simulink library "myLibrary"  (R2023a)
settings: Solver=VariableStepAuto  StartTime=0.0  StopTime=10.0  RelTol=1e-3
undefined symbols (not defined in the file): Cac_n1, ctrl1, Da, Discrete, dtha, ee_sli_rtmsupport, FA, gcbh, Ha, Ini, init_line, init_load, init_SG, init_TH, init_trafo, init_VSC, initMachineBlocks, Ka, Lf, Llkd_pu, Llkq1_pu, NET, P, plots_step, q0, Rac_n1, Radd, Rkd_pu, Rkq1_pu, Rload_add, sim_config, spsSteamTurbineModel, T_global, T_load, T_NET, T_SG, T_TH, T_trafo, T_VSC, Ts, tstep, V1
libraries: spsSeriesRLCBranchLib x57, spsParallelRLCBranchLib x39, eeGeneralControl x38, spsCurrentMeasurementLib x20, spsFirstOrderFilterLib x16, spsVoltageMeasurementLib x14, spsControlledVoltageSourceLib x12, $bdroot x9, dspsigops x6, spsThreePhaseVIMeasurementLib x5, spsPLL3phLib x4, spsThreePhaseBreakerLib x3
(part 6 of 7)

== system myLibrary/SG_step/Governor-Turbine/Steam Turbine and Governor/Model/4 mass shaft/2 masses ==
  note: Eeach block Mass implements discretized state-space equations
      | of the shaft mass dynamics using trapezoidal method.
      |
      | x(k)= Ad*x(k-1) + Bd*(u(k)+u(k-1))
      |
      | where:
      | x(k) =  State vector = [dw_n             deltat_n   ]'
      | u(k) =  Input vector = [(Ts_n+1 + Tt_n)  deltat_n-1 ]'
      | n    =  Mass number
      |
      | % Discrete state-space matrices
      | Ad = inv(In - Ts/2*A)*(In + Ts/2*A)
      | Bd = inv(In - Ts/2*A)*B*Ts/2
      |
      | where:
      | Continuous state-space matrices:
      | A=[ -K1*D  -K1*K
      |      K2     0   ];
      |
      | B=[ K1  K1*K
      |      0     0];
      |
      | In = eye(2,2)
      | K  = Rigidity (pu)
      | K1 =1/(2*H);  H= inertia  (pu)
      | K2 =N*pi/30;  N=nominal speed of sync. machine (rpm)
  note: Mass1 = generator rotor simulated in synchronous machine model
  Tt_5-2 : Inport
  dth_gen : Inport  Port=2
  Enable : EnablePort  PropagateVarSize=During execution
  Demux : Demux  Outputs=2
      settings: DisplayOption=none
  Ground : Ground
  Ground1 : Ground
  Mass2 : Subsystem  mask(Generic rotating mass){H=Ha(1), K=Ka(1), D=Da(1), dth0=dtha(1), N=N, Ts=Ts}
      mask prompts: H "Inertia H (pu)"; K "Rigidity K (pu):"; D "Damping D (pu):"; dth0 "Initial angle deviation delta_theta (rad):"; N "Nominal speed of synchronous machine (rpm):"; Ts "Sample time (s):"
      mask init: same as myLibrary/SG/Governor-Turbine/Steam Turbine and Governor/Model/4 mass shaft/1 mass/Mass2
  Mass3 : Subsystem  mask(Generic rotating mass){H=Ha(2), K=Ka(2), D=Da(2), dth0=dtha(2), N=N, Ts=Ts}
      mask prompts: H "Inertia H (pu)"; K "Rigidity K (pu):"; D "Damping D (pu):"; dth0 "Initial angle deviation delta_theta (rad):"; N "Nominal speed of synchronous machine (rpm):"; Ts "Sample time (s):"
      mask init: same as myLibrary/SG/Governor-Turbine/Steam Turbine and Governor/Model/4 mass shaft/1 mass/Mass2
  Mux : Mux  Inputs=[ 2 1 1 ]
  Mux1 : Mux  Inputs=[ 2 1 1 ]
  Selector : Selector  InputPortWidth=4  IndexOptions=Index vector (dialog)  Indices=[3 4]  OutputSizes=1
  Terminator : Terminator
  Ts_5-2 : Outport  InitialOutput=[0,0,0,0]
  dw_5-2 : Outport  Port=2  InitialOutput=[0,0,0,0]
  Tm_gen : Outport  Port=3
  wires:
  Mass2/3(dw) -> Mux1/3
  Mass3/3(dw) -> Mux1/2
  Mux1/1 -> dw_5-2/1
  Ground1/1 -> Mux1/1, Mux/1
  Demux/1 -> Mass3/2(Tt_n)
  Tt_5-2/1 -> Selector/1
  Selector/1 -> Demux/1
  Mux/1 -> Ts_5-2/1
  Mass3/2("Ts_n ") -> Mux/2, Mass2/1(Ts_n+1)
  Mass3/1(deltat_n) -> Terminator/1
  Ground/1 -> Mass3/1(Ts_n+1)
  Demux/2 -> Mass2/2(Tt_n)
  Mass2/1(deltat_n) -> Mass3/3(deltat_n-1)
  dth_gen/1 -> Mass2/3(deltat_n-1)
  Mass2/2("Ts_n ") -> Mux/3, Tm_gen/1

== system myLibrary/SG_step/Governor-Turbine/Steam Turbine and Governor/Model/4 mass shaft/3 masses ==
  note: Eeach block Mass implements discretized state-space equations
      | of the shaft mass dynamics using trapezoidal method.
      |
      | x(k)= Ad*x(k-1) + Bd*(u(k)+u(k-1))
      |
      | where:
      | x(k) =  State vector = [dw_n             deltat_n   ]'
      | u(k) =  Input vector = [(Ts_n+1 + Tt_n)  deltat_n-1 ]'
      | n    =  Mass number
      |
      | % Discrete state-space matrices
      | Ad = inv(In - Ts/2*A)*(In + Ts/2*A)
      | Bd = inv(In - Ts/2*A)*B*Ts/2
      |
      | where:
      | Continuous state-space matrices:
      | A=[ -K1*D  -K1*K
      |      K2     0   ];
      |
      | B=[ K1  K1*K
      |      0     0];
      |
      | In = eye(2,2)
      | K  = Rigidity (pu)
      | K1 =1/(2*H);  H= inertia  (pu)
      | K2 =N*pi/30;  N=nominal speed of sync. machine (rpm)
  note: Mass1 = generator rotor simulated in synchronous machine model
  Tt_5-2 : Inport
  dth_gen : Inport  Port=2
  Enable : EnablePort  PropagateVarSize=During execution
  Demux : Demux  Outputs=3
      settings: DisplayOption=none
  Ground : Ground
  Ground1 : Ground
  Mass2 : Subsystem  mask(Generic rotating mass){H=Ha(1), K=Ka(1), D=Da(1), dth0=dtha(1), N=N, Ts=Ts}
      mask prompts: H "Inertia H (pu)"; K "Rigidity K (pu):"; D "Damping D (pu):"; dth0 "Initial angle deviation delta_theta (rad):"; N "Nominal speed of synchronous machine (rpm):"; Ts "Sample time (s):"
      mask init: same as myLibrary/SG/Governor-Turbine/Steam Turbine and Governor/Model/4 mass shaft/1 mass/Mass2
  Mass3 : Subsystem  mask(Generic rotating mass){H=Ha(2), K=Ka(2), D=Da(2), dth0=dtha(2), N=N, Ts=Ts}
      mask prompts: H "Inertia H (pu)"; K "Rigidity K (pu):"; D "Damping D (pu):"; dth0 "Initial angle deviation delta_theta (rad):"; N "Nominal speed of synchronous machine (rpm):"; Ts "Sample time (s):"
      mask init: same as myLibrary/SG/Governor-Turbine/Steam Turbine and Governor/Model/4 mass shaft/1 mass/Mass2
  Mass4 : Subsystem  mask(Generic rotating mass){H=Ha(3), K=Ka(3), D=Da(3), dth0=dtha(3), N=N, Ts=Ts}
      mask prompts: H "Inertia H (pu)"; K "Rigidity K (pu):"; D "Damping D (pu):"; dth0 "Initial angle deviation delta_theta (rad):"; N "Nominal speed of synchronous machine (rpm):"; Ts "Sample time (s):"
      mask init: same as myLibrary/SG/Governor-Turbine/Steam Turbine and Governor/Model/4 mass shaft/1 mass/Mass2
  Mux : Mux
  Mux1 : Mux
  Selector : Selector  InputPortWidth=4  IndexOptions=Index vector (dialog)  Indices=[2 3 4]  OutputSizes=1
  Terminator : Terminator
  Ts_5-2 : Outport  InitialOutput=[0,0,0,0]
  dw_5-2 : Outport  Port=2  InitialOutput=[0,0,0,0]
  Tm_gen : Outport  Port=3
  wires:
  Mass2/3(dw) -> Mux1/4
  Mux1/1 -> dw_5-2/1
  Ground1/1 -> Mux1/1, Mux/1
  Mux/1 -> Ts_5-2/1
  Mass3/3(dw) -> Mux1/3
  Mass4/3(dw) -> Mux1/2
  Mass4/2("Ts_n ") -> Mux/2, Mass3/1(Ts_n+1)
  Mass3/1(deltat_n) -> Mass4/3(deltat_n-1)
  Mass2/1(deltat_n) -> Mass3/3(deltat_n-1)
  Demux/3 -> Mass2/2(Tt_n)
  Demux/2 -> Mass3/2(Tt_n)
  Demux/1 -> Mass4/2(Tt_n)
  Ground/1 -> Mass4/1(Ts_n+1)
  Mass4/1(deltat_n) -> Terminator/1
  dth_gen/1 -> Mass2/3(deltat_n-1)
  Mass2/2("Ts_n ") -> Tm_gen/1, Mux/4
  Selector/1 -> Demux/1
  Tt_5-2/1 -> Selector/1
  Mass3/2("Ts_n ") -> Mux/3, Mass2/1(Ts_n+1)

== system myLibrary/SG_step/Governor-Turbine/Steam Turbine and Governor/Model/4 mass shaft/4 masses ==
  note: Eeach block Mass implements discretized state-space equations
      | of the shaft mass dynamics using trapezoidal method.
      |
      | x(k)= Ad*x(k-1) + Bd*(u(k)+u(k-1))
      |
      | where:
      | x(k) =  State vector = [dw_n             deltat_n   ]'
      | u(k) =  Input vector = [(Ts_n+1 + Tt_n)  deltat_n-1 ]'
      | n    =  Mass number
      |
      | % Discrete state-space matrices
      | Ad = inv(In - Ts/2*A)*(In + Ts/2*A)
      | Bd = inv(In - Ts/2*A)*B*Ts/2
      |
      | where:
      | Continuous state-space matrices:
      | A=[ -K1*D  -K1*K
      |      K2     0   ];
      |
      | B=[ K1  K1*K
      |      0     0];
      |
      | In = eye(2,2)
      | K  = Rigidity (pu)
      | K1 =1/(2*H);  H= inertia  (pu)
      | K2 =N*pi/30;  N=nominal speed of sync. machine (rpm)
  note: Mass1 = generator rotor simulated in synchronous machine model
  Tt_5-2 : Inport
  dth_gen : Inport  Port=2
  Enable : EnablePort  PropagateVarSize=During execution
  Demux : Demux
      settings: DisplayOption=none
  Ground : Ground
  Mass2 : Subsystem  mask(Generic rotating mass){H=Ha(1), K=Ka(1), D=Da(1), dth0=initSG.delta2, N=N, Ts=Ts}
      mask prompts: H "Inertia H (pu)"; K "Rigidity K (pu):"; D "Damping D (pu):"; dth0 "Initial angle deviation delta_theta (rad):"; N "Nominal speed of synchronous machine (rpm):"; Ts "Sample time (s):"
      mask init: same as myLibrary/SG/Governor-Turbine/Steam Turbine and Governor/Model/4 mass shaft/1 mass/Mass2
  Mass3 : Subsystem  mask(Generic rotating mass){H=Ha(2), K=Ka(2), D=Da(2), dth0=initSG.delta3, N=N, Ts=Ts}
      mask prompts: H "Inertia H (pu)"; K "Rigidity K (pu):"; D "Damping D (pu):"; dth0 "Initial angle deviation delta_theta (rad):"; N "Nominal speed of synchronous machine (rpm):"; Ts "Sample time (s):"
      mask init: same as myLibrary/SG/Governor-Turbine/Steam Turbine and Governor/Model/4 mass shaft/1 mass/Mass2
  Mass4 : Subsystem  mask(Generic rotating mass){H=Ha(3), K=Ka(3), D=Da(3), dth0=initSG.delta4, N=N, Ts=Ts}
      mask prompts: H "Inertia H (pu)"; K "Rigidity K (pu):"; D "Damping D (pu):"; dth0 "Initial angle deviation delta_theta (rad):"; N "Nominal speed of synchronous machine (rpm):"; Ts "Sample time (s):"
      mask init: same as myLibrary/SG/Governor-Turbine/Steam Turbine and Governor/Model/4 mass shaft/1 mass/Mass2
  Mass5 : Subsystem  mask(Generic rotating mass){H=Ha(4), K=Ka(4), D=Da(4), dth0=initSG.delta5, N=N, Ts=Ts}
      mask prompts: H "Inertia H (pu)"; K "Rigidity K (pu):"; D "Damping D (pu):"; dth0 "Initial angle deviation delta_theta (rad):"; N "Nominal speed of synchronous machine (rpm):"; Ts "Sample time (s):"
      mask init: same as myLibrary/SG/Governor-Turbine/Steam Turbine and Governor/Model/4 mass shaft/1 mass/Mass2
  Mux : Mux
  Mux1 : Mux
  Terminator : Terminator
  Ts_5-2 : Outport  InitialOutput=[0,0,0,0]
  dw_5-2 : Outport  Port=2  InitialOutput=[0,0,0,0]
  Tm_gen : Outport  Port=3
  wires:
  Mass2/3(dw) -> Mux1/4
  Mass3/3(dw) -> Mux1/3
  Mux1/1 -> dw_5-2/1
  Mass4/3(dw) -> Mux1/2
  Mass5/3(dw) -> Mux1/1
  Mux/1 -> Ts_5-2/1
  Mass5/1(deltat_n) -> Terminator/1
  Ground/1 -> Mass5/1(Ts_n+1)
  Demux/1 -> Mass5/2(Tt_n)
  Demux/2 -> Mass4/2(Tt_n)
  Demux/3 -> Mass3/2(Tt_n)
  Demux/4 -> Mass2/2(Tt_n)
  Mass2/1(deltat_n) -> Mass3/3(deltat_n-1)
  Mass3/1(deltat_n) -> Mass4/3(deltat_n-1)
  Mass4/1(deltat_n) -> Mass5/3(deltat_n-1)
  Mass5/2("Ts_n ") -> Mux/1, Mass4/1(Ts_n+1)
  Mass4/2("Ts_n ") -> Mux/2, Mass3/1(Ts_n+1)
  Mass3/2("Ts_n ") -> Mux/3, Mass2/1(Ts_n+1)
  Tt_5-2/1 -> Demux/1
  dth_gen/1 -> Mass2/3(deltat_n-1)
  Mass2/2("Ts_n ") -> Mux/4, Tm_gen/1

== system myLibrary/SG_step/Governor-Turbine/Steam Turbine and Governor/Model/steam turbine MM/Stage 1 ==
  In1 : Inport
  Constant4 : Constant  Value=Ta(1)~=0  SampleTime=Ts
  Stage1 : Subsystem  TreatAsAtomicUnit=on
  Switch : Switch  Threshold=0.5  SaturateOnIntegerOverflow=off
  Out1 : Outport
  wires:
  Constant4/1 -> Stage1/Enable, Switch/2
  In1/1 -> Stage1/1(In1), Switch/3
  Stage1/1(Out1) -> Switch/1
  Switch/1 -> Out1/1

== system myLibrary/SG_step/Governor-Turbine/Steam Turbine and Governor/Model/steam turbine MM/Stage 2  ==
  In1 : Inport
  Constant3 : Constant  Value=Ta(2)~=0  SampleTime=Ts
  Stage2 : Subsystem  TreatAsAtomicUnit=on
  Switch1 : Switch  Threshold=0.5  SaturateOnIntegerOverflow=off
  Out1 : Outport
  wires:
  Stage2/1(Out1) -> Switch1/1
  Constant3/1 -> Stage2/Enable, Switch1/2
  Switch1/1 -> Out1/1
  In1/1 -> Stage2/1(In1), Switch1/3

== system myLibrary/SG_step/Governor-Turbine/Steam Turbine and Governor/Model/steam turbine MM/Stage 3 ==
  In1 : Inport
  Constant2 : Constant  Value=Ta(3)~=0  SampleTime=Ts
  Stage3 : Subsystem  TreatAsAtomicUnit=on
  Switch2 : Switch  Threshold=0.5  SaturateOnIntegerOverflow=off
  Out1 : Outport
  wires:
  Stage3/1(Out1) -> Switch2/1
  Constant2/1 -> Stage3/Enable, Switch2/2
  Switch2/1 -> Out1/1
  In1/1 -> Stage3/1(In1), Switch2/3

== system myLibrary/SG_step/Governor-Turbine/Steam Turbine and Governor/Model/steam turbine MM/Stage 4 ==
  In1 : Inport
  Constant1 : Constant  Value=Ta(4)~=0  SampleTime=Ts
  Stage4 : Subsystem  TreatAsAtomicUnit=on
  Switch3 : Switch  Threshold=0.5  SaturateOnIntegerOverflow=off
  Out1 : Outport
  wires:
  Stage4/1(Out1) -> Switch3/1
  Constant1/1 -> Stage4/Enable, Switch3/2
  In1/1 -> Stage4/1(In1), Switch3/3
  Switch3/1 -> Out1/1

== system myLibrary/SG/Governor-Turbine/Steam Turbine and Governor/Model/4 mass shaft/1 mass/Mass2 ==
  note: implements discretized state-space model of mass dynamic equations using trapezoidal method
      |
      | x(k)= Ad*x(k-1) + Bd*(u(k)+u(k-1))
  note: In order to avoid an algebraic loop
      | the deltat_n(k-1) value is sent to output 1
      | instead of  deltat_n(k).
      | The delay is then compensated by a
      | linear extrapolatiom (Prediction bloc)
  note: Initialization of this delay is not required
      | because x(k) is initialized by IC switch block
  Ts_n+1 : Inport
  Tt_n : Inport  Port=2
  deltat_n-1 : Inport  Port=3
  Ad*x(k-1) : Gain  Gain=Ad  Multiplication=Matrix(K*u)  SaturateOnIntegerOverflow=on  SampleTime=Ts  OutDataTypeStr=Inherit: Same as input  ParamDataTypeStr=Inherit: Same as input
  Bd*(u(k)+ u(k-1)) : Gain  Gain=Bd  Multiplication=Matrix(K*u)  SaturateOnIntegerOverflow=on  SampleTime=Ts  OutDataTypeStr=Inherit: Same as input  ParamDataTypeStr=Inherit: Same as input
  Delay_u : UnitDelay  SampleTime=Ts  HasFrameUpgradeWarning=on
  Delay_x : UnitDelay  InitialCondition=[0 dth0]  SampleTime=Ts  HasFrameUpgradeWarning=on
  Demux : Demux  Outputs=2
  Demux1 : Demux  Outputs=2
  Digital Clock : DigitalClock  SampleTime=Ts
  Gain11 : Gain  Gain=K  SaturateOnIntegerOverflow=on  OutDataTypeStr=Inherit: Same as input  ParamDataTypeStr=Inherit: Same as input
  IC : Switch  Threshold=Ts  SaturateOnIntegerOverflow=off  InputSameDT=off
  Mux : Mux  Inputs=2
  Prediction : Subsystem
  Sum1 : Sum  Inputs=+-  InputSameDT=on  SaturateOnIntegerOverflow=on  OutDataTypeStr=Inherit: Same as first input
  Sum3 : Sum  InputSameDT=on  SaturateOnIntegerOverflow=on  OutDataTypeStr=Inherit: Same as first input
  Sum9 : Sum  InputSameDT=on  SaturateOnIntegerOverflow=on  OutDataTypeStr=Inherit: Same as first input
  Terminator : Terminator
  sum : Sum  SaturateOnIntegerOverflow=on
  deltat_n : Outport  InitialOutput=0
  "Ts_n " : Outport  Port=2  InitialOutput=0
  dw : Outport  Port=3  InitialOutput=0
  wires:
  Prediction/1(O) -> deltat_n/1
  Demux1/1 -> Terminator/1
  Demux1/2 -> Prediction/1(I)
  Demux/2 -> Sum1/1  "x2(k)"
  Demux/1 -> dw/1  "x1(k)"
  IC/1 -> Demux/1, Delay_x/1
  Sum3/1 -> IC/1  "x(k)"
  Digital Clock/1 -> IC/2
  Delay_x/1 -> Ad*x(k-1)/1, Demux1/1, IC/3  "x(k-1)"
  Ad*x(k-1)/1 -> Sum3/1
  Bd*(u(k)+ u(k-1))/1 -> Sum3/2
  sum/1 -> Bd*(u(k)+ u(k-1))/1  "u(k) + u(k-1)"
  Delay_u/1 -> sum/2
  Tt_n/1 -> Sum9/2
  Ts_n+1/1 -> Sum9/1
  Sum9/1 -> Mux/1  "u1 (k)"
  deltat_n-1/1 -> Sum1/2, Mux/2  "u2(k)"
  Mux/1 -> sum/1, Delay_u/1  "u(k)"
  Sum1/1 -> Gain11/1
  Gain11/1 -> "Ts_n "/1

== system myLibrary/SG/Governor-Turbine/Steam Turbine and Governor/Model/4 mass shaft/2 masses/Mass2 ==
  note: Initialization of this delay is not required
      | because x(k) is initialized by IC switch block
  note: In order to avoid an algebraic loop
      | the deltat_n(k-1) value is sent to output 1
      | instead of  deltat_n(k).
      | The delay is then compensated by a
      | linear extrapolatiom (Prediction bloc)
  note: implements discretized state-space model of mass dynamic equations using trapezoidal method
      |
      | x(k)= Ad*x(k-1) + Bd*(u(k)+u(k-1))
  Ts_n+1 : Inport
  Tt_n : Inport  Port=2
  deltat_n-1 : Inport  Port=3
  Ad*x(k-1) : Gain  Gain=Ad  Multiplication=Matrix(K*u)  SaturateOnIntegerOverflow=on  SampleTime=Ts  OutDataTypeStr=Inherit: Same as input  ParamDataTypeStr=Inherit: Same as input
  Bd*(u(k)+ u(k-1)) : Gain  Gain=Bd  Multiplication=Matrix(K*u)  SaturateOnIntegerOverflow=on  SampleTime=Ts  OutDataTypeStr=Inherit: Same as input  ParamDataTypeStr=Inherit: Same as input
  Delay_u : UnitDelay  SampleTime=Ts  HasFrameUpgradeWarning=on
  Delay_x : UnitDelay  InitialCondition=[0 dth0]  SampleTime=Ts  HasFrameUpgradeWarning=on
  Demux : Demux  Outputs=2
  Demux1 : Demux  Outputs=2
  Digital Clock : DigitalClock  SampleTime=Ts
  Gain11 : Gain  Gain=K  SaturateOnIntegerOverflow=on  OutDataTypeStr=Inherit: Same as input  ParamDataTypeStr=Inherit: Same as input
  IC : Switch  Threshold=Ts  SaturateOnIntegerOverflow=off  InputSameDT=off
  Mux : Mux  Inputs=2
  Prediction : Subsystem
  Sum1 : Sum  Inputs=+-  InputSameDT=on  SaturateOnIntegerOverflow=on  OutDataTypeStr=Inherit: Same as first input
  Sum3 : Sum  InputSameDT=on  SaturateOnIntegerOverflow=on  OutDataTypeStr=Inherit: Same as first input
  Sum9 : Sum  InputSameDT=on  SaturateOnIntegerOverflow=on  OutDataTypeStr=Inherit: Same as first input
  Terminator : Terminator
  sum : Sum  SaturateOnIntegerOverflow=on
  deltat_n : Outport  InitialOutput=0
  "Ts_n " : Outport  Port=2  InitialOutput=0
  dw : Outport  Port=3  InitialOutput=0
  wires:
  Gain11/1 -> "Ts_n "/1
  Sum1/1 -> Gain11/1
  Mux/1 -> Delay_u/1, sum/1  "u(k)"
  deltat_n-1/1 -> Mux/2, Sum1/2  "u2(k)"
  Sum9/1 -> Mux/1  "u1 (k)"
  Ts_n+1/1 -> Sum9/1
  Tt_n/1 -> Sum9/2
  Delay_u/1 -> sum/2
  sum/1 -> Bd*(u(k)+ u(k-1))/1  "u(k) + u(k-1)"
  Bd*(u(k)+ u(k-1))/1 -> Sum3/2
  Ad*x(k-1)/1 -> Sum3/1
  Delay_x/1 -> IC/3, Demux1/1, Ad*x(k-1)/1  "x(k-1)"
  Digital Clock/1 -> IC/2
  Sum3/1 -> IC/1  "x(k)"
  IC/1 -> Delay_x/1, Demux/1
  Demux/1 -> dw/1  "x1(k)"
  Demux/2 -> Sum1/1  "x2(k)"
  Demux1/2 -> Prediction/1(I)
  Demux1/1 -> Terminator/1
  Prediction/1(O) -> deltat_n/1

== system myLibrary/SG/Governor-Turbine/Steam Turbine and Governor/Model/4 mass shaft/2 masses/Mass3 ==
  note: implements discretized state-space model of mass dynamic equations using trapezoidal method
      |
      | x(k)= Ad*x(k-1) + Bd*(u(k)+u(k-1))
  note: In order to avoid an algebraic loop
      | the deltat_n(k-1) value is sent to output 1
      | instead of  deltat_n(k).
      | The delay is then compensated by a
      | linear extrapolatiom (Prediction bloc)
  note: Initialization of this delay is not required
      | because x(k) is initialized by IC switch block
  Ts_n+1 : Inport
  Tt_n : Inport  Port=2
  deltat_n-1 : Inport  Port=3
  Ad*x(k-1) : Gain  Gain=Ad  Multiplication=Matrix(K*u)  SaturateOnIntegerOverflow=on  SampleTime=Ts  OutDataTypeStr=Inherit: Same as input  ParamDataTypeStr=Inherit: Same as input
  Bd*(u(k)+ u(k-1)) : Gain  Gain=Bd  Multiplication=Matrix(K*u)  SaturateOnIntegerOverflow=on  SampleTime=Ts  OutDataTypeStr=Inherit: Same as input  ParamDataTypeStr=Inherit: Same as input
  Delay_u : UnitDelay  SampleTime=Ts  HasFrameUpgradeWarning=on
  Delay_x : UnitDelay  InitialCondition=[0 dth0]  SampleTime=Ts  HasFrameUpgradeWarning=on
  Demux : Demux  Outputs=2
  Demux1 : Demux  Outputs=2
  Digital Clock : DigitalClock  SampleTime=Ts
  Gain11 : Gain  Gain=K  SaturateOnIntegerOverflow=on  OutDataTypeStr=Inherit: Same as input  ParamDataTypeStr=Inherit: Same as input
  IC : Switch  Threshold=Ts  SaturateOnIntegerOverflow=off  InputSameDT=off
  Mux : Mux  Inputs=2
  Prediction : Subsystem
  Sum1 : Sum  Inputs=+-  InputSameDT=on  SaturateOnIntegerOverflow=on  OutDataTypeStr=Inherit: Same as first input
  Sum3 : Sum  InputSameDT=on  SaturateOnIntegerOverflow=on  OutDataTypeStr=Inherit: Same as first input
  Sum9 : Sum  InputSameDT=on  SaturateOnIntegerOverflow=on  OutDataTypeStr=Inherit: Same as first input
  Terminator : Terminator
  sum : Sum  SaturateOnIntegerOverflow=on
  deltat_n : Outport  InitialOutput=0
  "Ts_n " : Outport  Port=2  InitialOutput=0
  dw : Outport  Port=3  InitialOutput=0
  wires:
  Prediction/1(O) -> deltat_n/1
  Demux1/1 -> Terminator/1
  Demux1/2 -> Prediction/1(I)
  Demux/2 -> Sum1/1  "x2(k)"
  Demux/1 -> dw/1  "x1(k)"
  IC/1 -> Demux/1, Delay_x/1
  Sum3/1 -> IC/1  "x(k)"
  Digital Clock/1 -> IC/2
  Delay_x/1 -> Ad*x(k-1)/1, Demux1/1, IC/3  "x(k-1)"
  Ad*x(k-1)/1 -> Sum3/1
  Bd*(u(k)+ u(k-1))/1 -> Sum3/2
  sum/1 -> Bd*(u(k)+ u(k-1))/1  "u(k) + u(k-1)"
  Delay_u/1 -> sum/2
  Tt_n/1 -> Sum9/2
  Ts_n+1/1 -> Sum9/1
  Sum9/1 -> Mux/1  "u1 (k)"
  deltat_n-1/1 -> Sum1/2, Mux/2  "u2(k)"
  Mux/1 -> sum/1, Delay_u/1  "u(k)"
  Sum1/1 -> Gain11/1
  Gain11/1 -> "Ts_n "/1

== system myLibrary/SG/Governor-Turbine/Steam Turbine and Governor/Model/4 mass shaft/3 masses/Mass2 ==
  note: implements discretized state-space model of mass dynamic equations using trapezoidal method
      |
      | x(k)= Ad*x(k-1) + Bd*(u(k)+u(k-1))
  note: In order to avoid an algebraic loop
      | the deltat_n(k-1) value is sent to output 1
      | instead of  deltat_n(k).
      | The delay is then compensated by a
      | linear extrapolatiom (Prediction bloc)
  note: Initialization of this delay is not required
      | because x(k) is initialized by IC switch block
  Ts_n+1 : Inport
  Tt_n : Inport  Port=2
  deltat_n-1 : Inport  Port=3
  Ad*x(k-1) : Gain  Gain=Ad  Multiplication=Matrix(K*u)  SaturateOnIntegerOverflow=on  SampleTime=Ts  OutDataTypeStr=Inherit: Same as input  ParamDataTypeStr=Inherit: Same as input
  Bd*(u(k)+ u(k-1)) : Gain  Gain=Bd  Multiplication=Matrix(K*u)  SaturateOnIntegerOverflow=on  SampleTime=Ts  OutDataTypeStr=Inherit: Same as input  ParamDataTypeStr=Inherit: Same as input
  Delay_u : UnitDelay  SampleTime=Ts  HasFrameUpgradeWarning=on
  Delay_x : UnitDelay  InitialCondition=[0 dth0]  SampleTime=Ts  HasFrameUpgradeWarning=on
  Demux : Demux  Outputs=2
  Demux1 : Demux  Outputs=2
  Digital Clock : DigitalClock  SampleTime=Ts
  Gain11 : Gain  Gain=K  SaturateOnIntegerOverflow=on  OutDataTypeStr=Inherit: Same as input  ParamDataTypeStr=Inherit: Same as input
  IC : Switch  Threshold=Ts  SaturateOnIntegerOverflow=off  InputSameDT=off
  Mux : Mux  Inputs=2
  Prediction : Subsystem
  Sum1 : Sum  Inputs=+-  InputSameDT=on  SaturateOnIntegerOverflow=on  OutDataTypeStr=Inherit: Same as first input
  Sum3 : Sum  InputSameDT=on  SaturateOnIntegerOverflow=on  OutDataTypeStr=Inherit: Same as first input
  Sum9 : Sum  InputSameDT=on  SaturateOnIntegerOverflow=on  OutDataTypeStr=Inherit: Same as first input
  Terminator : Terminator
  sum : Sum  SaturateOnIntegerOverflow=on
  deltat_n : Outport  InitialOutput=0
  "Ts_n " : Outport  Port=2  InitialOutput=0
  dw : Outport  Port=3  InitialOutput=0
  wires:
  Prediction/1(O) -> deltat_n/1
  Demux1/1 -> Terminator/1
  Demux1/2 -> Prediction/1(I)
  Demux/2 -> Sum1/1  "x2(k)"
  Demux/1 -> dw/1  "x1(k)"
  IC/1 -> Demux/1, Delay_x/1
  Sum3/1 -> IC/1  "x(k)"
  Digital Clock/1 -> IC/2
  Delay_x/1 -> Ad*x(k-1)/1, Demux1/1, IC/3  "x(k-1)"
  Ad*x(k-1)/1 -> Sum3/1
  Bd*(u(k)+ u(k-1))/1 -> Sum3/2
  sum/1 -> Bd*(u(k)+ u(k-1))/1  "u(k) + u(k-1)"
  Delay_u/1 -> sum/2
  Tt_n/1 -> Sum9/2
  Ts_n+1/1 -> Sum9/1
  Sum9/1 -> Mux/1  "u1 (k)"
  deltat_n-1/1 -> Sum1/2, Mux/2  "u2(k)"
  Mux/1 -> sum/1, Delay_u/1  "u(k)"
  Sum1/1 -> Gain11/1
  Gain11/1 -> "Ts_n "/1

== system myLibrary/SG/Governor-Turbine/Steam Turbine and Governor/Model/4 mass shaft/3 masses/Mass3 ==
  note: Initialization of this delay is not required
      | because x(k) is initialized by IC switch block
  note: In order to avoid an algebraic loop
      | the deltat_n(k-1) value is sent to output 1
      | instead of  deltat_n(k).
      | The delay is then compensated by a
      | linear extrapolatiom (Prediction bloc)
  note: implements discretized state-space model of mass dynamic equations using trapezoidal method
      |
      | x(k)= Ad*x(k-1) + Bd*(u(k)+u(k-1))
  Ts_n+1 : Inport
  Tt_n : Inport  Port=2
  deltat_n-1 : Inport  Port=3
  Ad*x(k-1) : Gain  Gain=Ad  Multiplication=Matrix(K*u)  SaturateOnIntegerOverflow=on  SampleTime=Ts  OutDataTypeStr=Inherit: Same as input  ParamDataTypeStr=Inherit: Same as input
  Bd*(u(k)+ u(k-1)) : Gain  Gain=Bd  Multiplication=Matrix(K*u)  SaturateOnIntegerOverflow=on  SampleTime=Ts  OutDataTypeStr=Inherit: Same as input  ParamDataTypeStr=Inherit: Same as input
  Delay_u : UnitDelay  SampleTime=Ts  HasFrameUpgradeWarning=on
  Delay_x : UnitDelay  InitialCondition=[0 dth0]  SampleTime=Ts  HasFrameUpgradeWarning=on
  Demux : Demux  Outputs=2
  Demux1 : Demux  Outputs=2
  Digital Clock : DigitalClock  SampleTime=Ts
  Gain11 : Gain  Gain=K  SaturateOnIntegerOverflow=on  OutDataTypeStr=Inherit: Same as input  ParamDataTypeStr=Inherit: Same as input
  IC : Switch  Threshold=Ts  SaturateOnIntegerOverflow=off  InputSameDT=off
  Mux : Mux  Inputs=2
  Prediction : Subsystem
  Sum1 : Sum  Inputs=+-  InputSameDT=on  SaturateOnIntegerOverflow=on  OutDataTypeStr=Inherit: Same as first input
  Sum3 : Sum  InputSameDT=on  SaturateOnIntegerOverflow=on  OutDataTypeStr=Inherit: Same as first input
  Sum9 : Sum  InputSameDT=on  SaturateOnIntegerOverflow=on  OutDataTypeStr=Inherit: Same as first input
  Terminator : Terminator
  sum : Sum  SaturateOnIntegerOverflow=on
  deltat_n : Outport  InitialOutput=0
  "Ts_n " : Outport  Port=2  InitialOutput=0
  dw : Outport  Port=3  InitialOutput=0
  wires:
  Gain11/1 -> "Ts_n "/1
  Sum1/1 -> Gain11/1
  Mux/1 -> Delay_u/1, sum/1  "u(k)"
  deltat_n-1/1 -> Mux/2, Sum1/2  "u2(k)"
  Sum9/1 -> Mux/1  "u1 (k)"
  Ts_n+1/1 -> Sum9/1
  Tt_n/1 -> Sum9/2
  Delay_u/1 -> sum/2
  sum/1 -> Bd*(u(k)+ u(k-1))/1  "u(k) + u(k-1)"
  Bd*(u(k)+ u(k-1))/1 -> Sum3/2
  Ad*x(k-1)/1 -> Sum3/1
  Delay_x/1 -> IC/3, Demux1/1, Ad*x(k-1)/1  "x(k-1)"
  Digital Clock/1 -> IC/2
  Sum3/1 -> IC/1  "x(k)"
  IC/1 -> Delay_x/1, Demux/1
  Demux/1 -> dw/1  "x1(k)"
  Demux/2 -> Sum1/1  "x2(k)"
  Demux1/2 -> Prediction/1(I)
  Demux1/1 -> Terminator/1
  Prediction/1(O) -> deltat_n/1

== system myLibrary/SG/Governor-Turbine/Steam Turbine and Governor/Model/4 mass shaft/3 masses/Mass4 ==
  note: implements discretized state-space model of mass dynamic equations using trapezoidal method
      |
      | x(k)= Ad*x(k-1) + Bd*(u(k)+u(k-1))
  note: In order to avoid an algebraic loop
      | the deltat_n(k-1) value is sent to output 1
      | instead of  deltat_n(k).
      | The delay is then compensated by a
      | linear extrapolatiom (Prediction bloc)
  note: Initialization of this delay is not required
      | because x(k) is initialized by IC switch block
  Ts_n+1 : Inport
  Tt_n : Inport  Port=2
  deltat_n-1 : Inport  Port=3
  Ad*x(k-1) : Gain  Gain=Ad  Multiplication=Matrix(K*u)  SaturateOnIntegerOverflow=on  SampleTime=Ts  OutDataTypeStr=Inherit: Same as input  ParamDataTypeStr=Inherit: Same as input
  Bd*(u(k)+ u(k-1)) : Gain  Gain=Bd  Multiplication=Matrix(K*u)  SaturateOnIntegerOverflow=on  SampleTime=Ts  OutDataTypeStr=Inherit: Same as input  ParamDataTypeStr=Inherit: Same as input
  Delay_u : UnitDelay  SampleTime=Ts  HasFrameUpgradeWarning=on
  Delay_x : UnitDelay  InitialCondition=[0 dth0]  SampleTime=Ts  HasFrameUpgradeWarning=on
  Demux : Demux  Outputs=2
  Demux1 : Demux  Outputs=2
  Digital Clock : DigitalClock  SampleTime=Ts
  Gain11 : Gain  Gain=K  SaturateOnIntegerOverflow=on  OutDataTypeStr=Inherit: Same as input  ParamDataTypeStr=Inherit: Same as input
  IC : Switch  Threshold=Ts  SaturateOnIntegerOverflow=off  InputSameDT=off
  Mux : Mux  Inputs=2
  Prediction : Subsystem
  Sum1 : Sum  Inputs=+-  InputSameDT=on  SaturateOnIntegerOverflow=on  OutDataTypeStr=Inherit: Same as first input
  Sum3 : Sum  InputSameDT=on  SaturateOnIntegerOverflow=on  OutDataTypeStr=Inherit: Same as first input
  Sum9 : Sum  InputSameDT=on  SaturateOnIntegerOverflow=on  OutDataTypeStr=Inherit: Same as first input
  Terminator : Terminator
  sum : Sum  SaturateOnIntegerOverflow=on
  deltat_n : Outport  InitialOutput=0
  "Ts_n " : Outport  Port=2  InitialOutput=0
  dw : Outport  Port=3  InitialOutput=0
  wires:
  Prediction/1(O) -> deltat_n/1
  Demux1/1 -> Terminator/1
  Demux1/2 -> Prediction/1(I)
  Demux/2 -> Sum1/1  "x2(k)"
  Demux/1 -> dw/1  "x1(k)"
  IC/1 -> Demux/1, Delay_x/1
  Sum3/1 -> IC/1  "x(k)"
  Digital Clock/1 -> IC/2
  Delay_x/1 -> Ad*x(k-1)/1, Demux1/1, IC/3  "x(k-1)"
  Ad*x(k-1)/1 -> Sum3/1
  Bd*(u(k)+ u(k-1))/1 -> Sum3/2
  sum/1 -> Bd*(u(k)+ u(k-1))/1  "u(k) + u(k-1)"
  Delay_u/1 -> sum/2
  Tt_n/1 -> Sum9/2
  Ts_n+1/1 -> Sum9/1
  Sum9/1 -> Mux/1  "u1 (k)"
  deltat_n-1/1 -> Sum1/2, Mux/2  "u2(k)"
  Mux/1 -> sum/1, Delay_u/1  "u(k)"
  Sum1/1 -> Gain11/1
  Gain11/1 -> "Ts_n "/1

== system myLibrary/SG/Governor-Turbine/Steam Turbine and Governor/Model/4 mass shaft/4 masses/Mass2 ==
  note: Initialization of this delay is not required
      | because x(k) is initialized by IC switch block
  note: In order to avoid an algebraic loop
      | the deltat_n(k-1) value is sent to output 1
      | instead of  deltat_n(k).
      | The delay is then compensated by a
      | linear extrapolatiom (Prediction bloc)
  note: implements discretized state-space model of mass dynamic equations using trapezoidal method
      |
      | x(k)= Ad*x(k-1) + Bd*(u(k)+u(k-1))
  Ts_n+1 : Inport
  Tt_n : Inport  Port=2
  deltat_n-1 : Inport  Port=3
  Ad*x(k-1) : Gain  Gain=Ad  Multiplication=Matrix(K*u)  SaturateOnIntegerOverflow=on  SampleTime=Ts  OutDataTypeStr=Inherit: Same as input  ParamDataTypeStr=Inherit: Same as input
  Bd*(u(k)+ u(k-1)) : Gain  Gain=Bd  Multiplication=Matrix(K*u)  SaturateOnIntegerOverflow=on  SampleTime=Ts  OutDataTypeStr=Inherit: Same as input  ParamDataTypeStr=Inherit: Same as input
  Delay_u : UnitDelay  SampleTime=Ts  HasFrameUpgradeWarning=on
  Delay_x : UnitDelay  InitialCondition=[0 initSG.delta2]  SampleTime=Ts  HasFrameUpgradeWarning=on
  Demux : Demux  Outputs=2
  Demux1 : Demux  Outputs=2
  Digital Clock : DigitalClock  SampleTime=Ts
  Gain11 : Gain  Gain=K  SaturateOnIntegerOverflow=on  OutDataTypeStr=Inherit: Same as input  ParamDataTypeStr=Inherit: Same as input
  IC : Switch  Threshold=Ts  SaturateOnIntegerOverflow=off  InputSameDT=off
  Mux : Mux  Inputs=2
  Prediction : Subsystem
  Sum1 : Sum  Inputs=+-  InputSameDT=on  SaturateOnIntegerOverflow=on  OutDataTypeStr=Inherit: Same as first input
  Sum3 : Sum  InputSameDT=on  SaturateOnIntegerOverflow=on  OutDataTypeStr=Inherit: Same as first input
  Sum9 : Sum  InputSameDT=on  SaturateOnIntegerOverflow=on  OutDataTypeStr=Inherit: Same as first input
  Terminator : Terminator
  sum : Sum  SaturateOnIntegerOverflow=on
  deltat_n : Outport  InitialOutput=0
  "Ts_n " : Outport  Port=2  InitialOutput=0
  dw : Outport  Port=3  InitialOutput=0
  wires:
  Gain11/1 -> "Ts_n "/1
  Sum1/1 -> Gain11/1
  Mux/1 -> Delay_u/1, sum/1  "u(k)"
  deltat_n-1/1 -> Mux/2, Sum1/2  "u2(k)"
  Sum9/1 -> Mux/1  "u1 (k)"
  Ts_n+1/1 -> Sum9/1
  Tt_n/1 -> Sum9/2
  Delay_u/1 -> sum/2
  sum/1 -> Bd*(u(k)+ u(k-1))/1  "u(k) + u(k-1)"
  Bd*(u(k)+ u(k-1))/1 -> Sum3/2
  Ad*x(k-1)/1 -> Sum3/1
  Delay_x/1 -> IC/3, Demux1/1, Ad*x(k-1)/1  "x(k-1)"
  Digital Clock/1 -> IC/2
  Sum3/1 -> IC/1  "x(k)"
  IC/1 -> Delay_x/1, Demux/1
  Demux/1 -> dw/1  "x1(k)"
  Demux/2 -> Sum1/1  "x2(k)"
  Demux1/2 -> Prediction/1(I)
  Demux1/1 -> Terminator/1
  Prediction/1(O) -> deltat_n/1

== system myLibrary/SG/Governor-Turbine/Steam Turbine and Governor/Model/4 mass shaft/4 masses/Mass3 ==
  note: implements discretized state-space model of mass dynamic equations using trapezoidal method
      |
      | x(k)= Ad*x(k-1) + Bd*(u(k)+u(k-1))
  note: In order to avoid an algebraic loop
      | the deltat_n(k-1) value is sent to output 1
      | instead of  deltat_n(k).
      | The delay is then compensated by a
      | linear extrapolatiom (Prediction bloc)
  note: Initialization of this delay is not required
      | because x(k) is initialized by IC switch block
  Ts_n+1 : Inport
  Tt_n : Inport  Port=2
  deltat_n-1 : Inport  Port=3
  Ad*x(k-1) : Gain  Gain=Ad  Multiplication=Matrix(K*u)  SaturateOnIntegerOverflow=on  SampleTime=Ts  OutDataTypeStr=Inherit: Same as input  ParamDataTypeStr=Inherit: Same as input
  Bd*(u(k)+ u(k-1)) : Gain  Gain=Bd  Multiplication=Matrix(K*u)  SaturateOnIntegerOverflow=on  SampleTime=Ts  OutDataTypeStr=Inherit: Same as input  ParamDataTypeStr=Inherit: Same as input
  Delay_u : UnitDelay  SampleTime=Ts  HasFrameUpgradeWarning=on
  Delay_x : UnitDelay  InitialCondition=[0 initSG.delta3]  SampleTime=Ts  HasFrameUpgradeWarning=on
  Demux : Demux  Outputs=2
  Demux1 : Demux  Outputs=2
  Digital Clock : DigitalClock  SampleTime=Ts
  Gain11 : Gain  Gain=K  SaturateOnIntegerOverflow=on  OutDataTypeStr=Inherit: Same as input  ParamDataTypeStr=Inherit: Same as input
  IC : Switch  Threshold=Ts  SaturateOnIntegerOverflow=off  InputSameDT=off
  Mux : Mux  Inputs=2
  Prediction : Subsystem
  Sum1 : Sum  Inputs=+-  InputSameDT=on  SaturateOnIntegerOverflow=on  OutDataTypeStr=Inherit: Same as first input
  Sum3 : Sum  InputSameDT=on  SaturateOnIntegerOverflow=on  OutDataTypeStr=Inherit: Same as first input
  Sum9 : Sum  InputSameDT=on  SaturateOnIntegerOverflow=on  OutDataTypeStr=Inherit: Same as first input
  Terminator : Terminator
  sum : Sum  SaturateOnIntegerOverflow=on
  deltat_n : Outport  InitialOutput=0
  "Ts_n " : Outport  Port=2  InitialOutput=0
  dw : Outport  Port=3  InitialOutput=0
  wires:
  Prediction/1(O) -> deltat_n/1
  Demux1/1 -> Terminator/1
  Demux1/2 -> Prediction/1(I)
  Demux/2 -> Sum1/1  "x2(k)"
  Demux/1 -> dw/1  "x1(k)"
  IC/1 -> Demux/1, Delay_x/1
  Sum3/1 -> IC/1  "x(k)"
  Digital Clock/1 -> IC/2
  Delay_x/1 -> Ad*x(k-1)/1, Demux1/1, IC/3  "x(k-1)"
  Ad*x(k-1)/1 -> Sum3/1
  Bd*(u(k)+ u(k-1))/1 -> Sum3/2
  sum/1 -> Bd*(u(k)+ u(k-1))/1  "u(k) + u(k-1)"
  Delay_u/1 -> sum/2
  Tt_n/1 -> Sum9/2
  Ts_n+1/1 -> Sum9/1
  Sum9/1 -> Mux/1  "u1 (k)"
  deltat_n-1/1 -> Sum1/2, Mux/2  "u2(k)"
  Mux/1 -> sum/1, Delay_u/1  "u(k)"
  Sum1/1 -> Gain11/1
  Gain11/1 -> "Ts_n "/1

== system myLibrary/SG/Governor-Turbine/Steam Turbine and Governor/Model/4 mass shaft/4 masses/Mass4 ==
  note: Initialization of this delay is not required
      | because x(k) is initialized by IC switch block
  note: In order to avoid an algebraic loop
      | the deltat_n(k-1) value is sent to output 1
      | instead of  deltat_n(k).
      | The delay is then compensated by a
      | linear extrapolatiom (Prediction bloc)
  note: implements discretized state-space model of mass dynamic equations using trapezoidal method
      |
      | x(k)= Ad*x(k-1) + Bd*(u(k)+u(k-1))
  Ts_n+1 : Inport
  Tt_n : Inport  Port=2
  deltat_n-1 : Inport  Port=3
  Ad*x(k-1) : Gain  Gain=Ad  Multiplication=Matrix(K*u)  SaturateOnIntegerOverflow=on  SampleTime=Ts  OutDataTypeStr=Inherit: Same as input  ParamDataTypeStr=Inherit: Same as input
  Bd*(u(k)+ u(k-1)) : Gain  Gain=Bd  Multiplication=Matrix(K*u)  SaturateOnIntegerOverflow=on  SampleTime=Ts  OutDataTypeStr=Inherit: Same as input  ParamDataTypeStr=Inherit: Same as input
  Delay_u : UnitDelay  SampleTime=Ts  HasFrameUpgradeWarning=on
  Delay_x : UnitDelay  InitialCondition=[0 initSG.delta4]  SampleTime=Ts  HasFrameUpgradeWarning=on
  Demux : Demux  Outputs=2
  Demux1 : Demux  Outputs=2
  Digital Clock : DigitalClock  SampleTime=Ts
  Gain11 : Gain  Gain=K  SaturateOnIntegerOverflow=on  OutDataTypeStr=Inherit: Same as input  ParamDataTypeStr=Inherit: Same as input
  IC : Switch  Threshold=Ts  SaturateOnIntegerOverflow=off  InputSameDT=off
  Mux : Mux  Inputs=2
  Prediction : Subsystem
  Sum1 : Sum  Inputs=+-  InputSameDT=on  SaturateOnIntegerOverflow=on  OutDataTypeStr=Inherit: Same as first input
  Sum3 : Sum  InputSameDT=on  SaturateOnIntegerOverflow=on  OutDataTypeStr=Inherit: Same as first input
  Sum9 : Sum  InputSameDT=on  SaturateOnIntegerOverflow=on  OutDataTypeStr=Inherit: Same as first input
  Terminator : Terminator
  sum : Sum  SaturateOnIntegerOverflow=on
  deltat_n : Outport  InitialOutput=0
  "Ts_n " : Outport  Port=2  InitialOutput=0
  dw : Outport  Port=3  InitialOutput=0
  wires:
  Gain11/1 -> "Ts_n "/1
  Sum1/1 -> Gain11/1
  Mux/1 -> Delay_u/1, sum/1  "u(k)"
  deltat_n-1/1 -> Mux/2, Sum1/2  "u2(k)"
  Sum9/1 -> Mux/1  "u1 (k)"
  Ts_n+1/1 -> Sum9/1
  Tt_n/1 -> Sum9/2
  Delay_u/1 -> sum/2
  sum/1 -> Bd*(u(k)+ u(k-1))/1  "u(k) + u(k-1)"
  Bd*(u(k)+ u(k-1))/1 -> Sum3/2
  Ad*x(k-1)/1 -> Sum3/1
  Delay_x/1 -> IC/3, Demux1/1, Ad*x(k-1)/1  "x(k-1)"
  Digital Clock/1 -> IC/2
  Sum3/1 -> IC/1  "x(k)"
  IC/1 -> Delay_x/1, Demux/1
  Demux/1 -> dw/1  "x1(k)"
  Demux/2 -> Sum1/1  "x2(k)"
  Demux1/2 -> Prediction/1(I)
  Demux1/1 -> Terminator/1
  Prediction/1(O) -> deltat_n/1

== system myLibrary/SG/Governor-Turbine/Steam Turbine and Governor/Model/4 mass shaft/4 masses/Mass5 ==
  note: implements discretized state-space model of mass dynamic equations using trapezoidal method
      |
      | x(k)= Ad*x(k-1) + Bd*(u(k)+u(k-1))
  note: In order to avoid an algebraic loop
      | the deltat_n(k-1) value is sent to output 1
      | instead of  deltat_n(k).
      | The delay is then compensated by a
      | linear extrapolatiom (Prediction bloc)
  note: Initialization of this delay is not required
      | because x(k) is initialized by IC switch block
  Ts_n+1 : Inport
  Tt_n : Inport  Port=2
  deltat_n-1 : Inport  Port=3
  Ad*x(k-1) : Gain  Gain=Ad  Multiplication=Matrix(K*u)  SaturateOnIntegerOverflow=on  SampleTime=Ts  OutDataTypeStr=Inherit: Same as input  ParamDataTypeStr=Inherit: Same as input
  Bd*(u(k)+ u(k-1)) : Gain  Gain=Bd  Multiplication=Matrix(K*u)  SaturateOnIntegerOverflow=on  SampleTime=Ts  OutDataTypeStr=Inherit: Same as input  ParamDataTypeStr=Inherit: Same as input
  Delay_u : UnitDelay  SampleTime=Ts  HasFrameUpgradeWarning=on
  Delay_x : UnitDelay  InitialCondition=[0 initSG.delta5]  SampleTime=Ts  HasFrameUpgradeWarning=on
  Demux : Demux  Outputs=2
  Demux1 : Demux  Outputs=2
  Digital Clock : DigitalClock  SampleTime=Ts
  Gain11 : Gain  Gain=K  SaturateOnIntegerOverflow=on  OutDataTypeStr=Inherit: Same as input  ParamDataTypeStr=Inherit: Same as input
  IC : Switch  Threshold=Ts  SaturateOnIntegerOverflow=off  InputSameDT=off
  Mux : Mux  Inputs=2
  Prediction : Subsystem
  Sum1 : Sum  Inputs=+-  InputSameDT=on  SaturateOnIntegerOverflow=on  OutDataTypeStr=Inherit: Same as first input
  Sum3 : Sum  InputSameDT=on  SaturateOnIntegerOverflow=on  OutDataTypeStr=Inherit: Same as first input
  Sum9 : Sum  InputSameDT=on  SaturateOnIntegerOverflow=on  OutDataTypeStr=Inherit: Same as first input
  Terminator : Terminator
  sum : Sum  SaturateOnIntegerOverflow=on
  deltat_n : Outport  InitialOutput=0
  "Ts_n " : Outport  Port=2  InitialOutput=0
  dw : Outport  Port=3  InitialOutput=0
  wires:
  Prediction/1(O) -> deltat_n/1
  Demux1/1 -> Terminator/1
  Demux1/2 -> Prediction/1(I)
  Demux/2 -> Sum1/1  "x2(k)"
  Demux/1 -> dw/1  "x1(k)"
  IC/1 -> Demux/1, Delay_x/1
  Sum3/1 -> IC/1  "x(k)"
  Digital Clock/1 -> IC/2
  Delay_x/1 -> Ad*x(k-1)/1, Demux1/1, IC/3  "x(k-1)"
  Ad*x(k-1)/1 -> Sum3/1
  Bd*(u(k)+ u(k-1))/1 -> Sum3/2
  sum/1 -> Bd*(u(k)+ u(k-1))/1  "u(k) + u(k-1)"
  Delay_u/1 -> sum/2
  Tt_n/1 -> Sum9/2
  Ts_n+1/1 -> Sum9/1
  Sum9/1 -> Mux/1  "u1 (k)"
  deltat_n-1/1 -> Sum1/2, Mux/2  "u2(k)"
  Mux/1 -> sum/1, Delay_u/1  "u(k)"
  Sum1/1 -> Gain11/1
  Gain11/1 -> "Ts_n "/1

== system myLibrary/SG/Governor-Turbine/Steam Turbine and Governor/Model/steam turbine MM/Stage 1/Stage1 ==
  In1 : Inport
  Enable : EnablePort
  Stage1 : spsFirstOrderFilterLib/First-Order Filter  FilterType=Lowpass  Tc=T1  Ts=Ts  Initialize=on  Vac_Init=[0, 0, 60]  Vdc_Init=f0  PlotResponse=off  FreqRange="[0,  200,  1]"
  Out1 : Outport  OutputWhenDisabled=reset  InitialOutput=0
  wires:
  In1/1 -> Stage1/1
  Stage1/1 -> Out1/1

== system myLibrary/SG/Governor-Turbine/Steam Turbine and Governor/Model/steam turbine MM/Stage 2 /Stage2 ==
  In1 : Inport
  Enable : EnablePort
  Stage2 : spsFirstOrderFilterLib/First-Order Filter  FilterType=Lowpass  Tc=T2  Ts=Ts  Initialize=on  Vac_Init=[0, 0, 60]  Vdc_Init=f0  PlotResponse=off  FreqRange="[0,  200,  1]"
  Out1 : Outport  OutputWhenDisabled=reset  InitialOutput=0
  wires:
  Stage2/1 -> Out1/1
  In1/1 -> Stage2/1

== system myLibrary/SG/Governor-Turbine/Steam Turbine and Governor/Model/steam turbine MM/Stage 3/Stage3 ==
  In1 : Inport
  Enable : EnablePort
  Stage3 : spsFirstOrderFilterLib/First-Order Filter  FilterType=Lowpass  Tc=T3  Ts=Ts  Initialize=on  Vac_Init=[0, 0, 60]  Vdc_Init=f0  PlotResponse=off  FreqRange="[0,  200,  1]"
  Out1 : Outport  OutputWhenDisabled=reset  InitialOutput=0
  wires:
  In1/1 -> Stage3/1
  Stage3/1 -> Out1/1

== system myLibrary/SG/Governor-Turbine/Steam Turbine and Governor/Model/steam turbine MM/Stage 4/Stage4 ==
  In1 : Inport
  Enable : EnablePort
  Stage4 : spsFirstOrderFilterLib/First-Order Filter  FilterType=Lowpass  Tc=T4  Ts=Ts  Initialize=on  Vac_Init=[0, 0, 60]  Vdc_Init=f0  PlotResponse=off  FreqRange="[0,  200,  1]"
  Out1 : Outport  OutputWhenDisabled=reset  InitialOutput=0
  wires:
  Stage4/1 -> Out1/1
  In1/1 -> Stage4/1

== system myLibrary/SG_step/Governor-Turbine/Steam Turbine and Governor/Model/4 mass shaft/1 mass/Mass2 ==
  note: implements discretized state-space model of mass dynamic equations using trapezoidal method
      |
      | x(k)= Ad*x(k-1) + Bd*(u(k)+u(k-1))
  note: In order to avoid an algebraic loop
      | the deltat_n(k-1) value is sent to output 1
      | instead of  deltat_n(k).
      | The delay is then compensated by a
      | linear extrapolatiom (Prediction bloc)
  note: Initialization of this delay is not required
      | because x(k) is initialized by IC switch block
  Ts_n+1 : Inport
  Tt_n : Inport  Port=2
  deltat_n-1 : Inport  Port=3
  Ad*x(k-1) : Gain  Gain=Ad  Multiplication=Matrix(K*u)  SaturateOnIntegerOverflow=on  SampleTime=Ts  OutDataTypeStr=Inherit: Same as input  ParamDataTypeStr=Inherit: Same as input
  Bd*(u(k)+ u(k-1)) : Gain  Gain=Bd  Multiplication=Matrix(K*u)  SaturateOnIntegerOverflow=on  SampleTime=Ts  OutDataTypeStr=Inherit: Same as input  ParamDataTypeStr=Inherit: Same as input
  Delay_u : UnitDelay  SampleTime=Ts  HasFrameUpgradeWarning=on
  Delay_x : UnitDelay  InitialCondition=[0 dth0]  SampleTime=Ts  HasFrameUpgradeWarning=on
  Demux : Demux  Outputs=2
  Demux1 : Demux  Outputs=2
  Digital Clock : DigitalClock  SampleTime=Ts
  Gain11 : Gain  Gain=K  SaturateOnIntegerOverflow=on  OutDataTypeStr=Inherit: Same as input  ParamDataTypeStr=Inherit: Same as input
  IC : Switch  Threshold=Ts  SaturateOnIntegerOverflow=off  InputSameDT=off
  Mux : Mux  Inputs=2
  Prediction : Subsystem
  Sum1 : Sum  Inputs=+-  InputSameDT=on  SaturateOnIntegerOverflow=on  OutDataTypeStr=Inherit: Same as first input
  Sum3 : Sum  InputSameDT=on  SaturateOnIntegerOverflow=on  OutDataTypeStr=Inherit: Same as first input
  Sum9 : Sum  InputSameDT=on  SaturateOnIntegerOverflow=on  OutDataTypeStr=Inherit: Same as first input
  Terminator : Terminator
  sum : Sum  SaturateOnIntegerOverflow=on
  deltat_n : Outport  InitialOutput=0
  "Ts_n " : Outport  Port=2  InitialOutput=0
  dw : Outport  Port=3  InitialOutput=0
  wires:
  Prediction/1(O) -> deltat_n/1
  Demux1/1 -> Terminator/1
  Demux1/2 -> Prediction/1(I)
  Demux/2 -> Sum1/1  "x2(k)"
  Demux/1 -> dw/1  "x1(k)"
  IC/1 -> Demux/1, Delay_x/1
  Sum3/1 -> IC/1  "x(k)"
  Digital Clock/1 -> IC/2
  Delay_x/1 -> Ad*x(k-1)/1, Demux1/1, IC/3  "x(k-1)"
  Ad*x(k-1)/1 -> Sum3/1
  Bd*(u(k)+ u(k-1))/1 -> Sum3/2
  sum/1 -> Bd*(u(k)+ u(k-1))/1  "u(k) + u(k-1)"
  Delay_u/1 -> sum/2
  Tt_n/1 -> Sum9/2
  Ts_n+1/1 -> Sum9/1
  Sum9/1 -> Mux/1  "u1 (k)"
  deltat_n-1/1 -> Sum1/2, Mux/2  "u2(k)"
  Mux/1 -> sum/1, Delay_u/1  "u(k)"
  Sum1/1 -> Gain11/1
  Gain11/1 -> "Ts_n "/1

== system myLibrary/SG_step/Governor-Turbine/Steam Turbine and Governor/Model/4 mass shaft/2 masses/Mass2 ==
  note: Initialization of this delay is not required
      | because x(k) is initialized by IC switch block
  note: In order to avoid an algebraic loop
      | the deltat_n(k-1) value is sent to output 1
      | instead of  deltat_n(k).
      | The delay is then compensated by a
      | linear extrapolatiom (Prediction bloc)
  note: implements discretized state-space model of mass dynamic equations using trapezoidal method
      |
      | x(k)= Ad*x(k-1) + Bd*(u(k)+u(k-1))
  Ts_n+1 : Inport
  Tt_n : Inport  Port=2
  deltat_n-1 : Inport  Port=3
  Ad*x(k-1) : Gain  Gain=Ad  Multiplication=Matrix(K*u)  SaturateOnIntegerOverflow=on  SampleTime=Ts  OutDataTypeStr=Inherit: Same as input  ParamDataTypeStr=Inherit: Same as input
  Bd*(u(k)+ u(k-1)) : Gain  Gain=Bd  Multiplication=Matrix(K*u)  SaturateOnIntegerOverflow=on  SampleTime=Ts  OutDataTypeStr=Inherit: Same as input  ParamDataTypeStr=Inherit: Same as input
  Delay_u : UnitDelay  SampleTime=Ts  HasFrameUpgradeWarning=on
  Delay_x : UnitDelay  InitialCondition=[0 dth0]  SampleTime=Ts  HasFrameUpgradeWarning=on
  Demux : Demux  Outputs=2
  Demux1 : Demux  Outputs=2
  Digital Clock : DigitalClock  SampleTime=Ts
  Gain11 : Gain  Gain=K  SaturateOnIntegerOverflow=on  OutDataTypeStr=Inherit: Same as input  ParamDataTypeStr=Inherit: Same as input
  IC : Switch  Threshold=Ts  SaturateOnIntegerOverflow=off  InputSameDT=off
  Mux : Mux  Inputs=2
  Prediction : Subsystem
  Sum1 : Sum  Inputs=+-  InputSameDT=on  SaturateOnIntegerOverflow=on  OutDataTypeStr=Inherit: Same as first input
  Sum3 : Sum  InputSameDT=on  SaturateOnIntegerOverflow=on  OutDataTypeStr=Inherit: Same as first input
  Sum9 : Sum  InputSameDT=on  SaturateOnIntegerOverflow=on  OutDataTypeStr=Inherit: Same as first input
  Terminator : Terminator
  sum : Sum  SaturateOnIntegerOverflow=on
  deltat_n : Outport  InitialOutput=0
  "Ts_n " : Outport  Port=2  InitialOutput=0
  dw : Outport  Port=3  InitialOutput=0
  wires:
  Gain11/1 -> "Ts_n "/1
  Sum1/1 -> Gain11/1
  Mux/1 -> Delay_u/1, sum/1  "u(k)"
  deltat_n-1/1 -> Mux/2, Sum1/2  "u2(k)"
  Sum9/1 -> Mux/1  "u1 (k)"
  Ts_n+1/1 -> Sum9/1
  Tt_n/1 -> Sum9/2
  Delay_u/1 -> sum/2
  sum/1 -> Bd*(u(k)+ u(k-1))/1  "u(k) + u(k-1)"
  Bd*(u(k)+ u(k-1))/1 -> Sum3/2
  Ad*x(k-1)/1 -> Sum3/1
  Delay_x/1 -> IC/3, Demux1/1, Ad*x(k-1)/1  "x(k-1)"
  Digital Clock/1 -> IC/2
  Sum3/1 -> IC/1  "x(k)"
  IC/1 -> Delay_x/1, Demux/1
  Demux/1 -> dw/1  "x1(k)"
  Demux/2 -> Sum1/1  "x2(k)"
  Demux1/2 -> Prediction/1(I)
  Demux1/1 -> Terminator/1
  Prediction/1(O) -> deltat_n/1

== system myLibrary/SG_step/Governor-Turbine/Steam Turbine and Governor/Model/4 mass shaft/2 masses/Mass3 ==
  note: implements discretized state-space model of mass dynamic equations using trapezoidal method
      |
      | x(k)= Ad*x(k-1) + Bd*(u(k)+u(k-1))
  note: In order to avoid an algebraic loop
      | the deltat_n(k-1) value is sent to output 1
      | instead of  deltat_n(k).
      | The delay is then compensated by a
      | linear extrapolatiom (Prediction bloc)
  note: Initialization of this delay is not required
      | because x(k) is initialized by IC switch block
  Ts_n+1 : Inport
  Tt_n : Inport  Port=2
  deltat_n-1 : Inport  Port=3
  Ad*x(k-1) : Gain  Gain=Ad  Multiplication=Matrix(K*u)  SaturateOnIntegerOverflow=on  SampleTime=Ts  OutDataTypeStr=Inherit: Same as input  ParamDataTypeStr=Inherit: Same as input
  Bd*(u(k)+ u(k-1)) : Gain  Gain=Bd  Multiplication=Matrix(K*u)  SaturateOnIntegerOverflow=on  SampleTime=Ts  OutDataTypeStr=Inherit: Same as input  ParamDataTypeStr=Inherit: Same as input
  Delay_u : UnitDelay  SampleTime=Ts  HasFrameUpgradeWarning=on
  Delay_x : UnitDelay  InitialCondition=[0 dth0]  SampleTime=Ts  HasFrameUpgradeWarning=on
  Demux : Demux  Outputs=2
  Demux1 : Demux  Outputs=2
  Digital Clock : DigitalClock  SampleTime=Ts
  Gain11 : Gain  Gain=K  SaturateOnIntegerOverflow=on  OutDataTypeStr=Inherit: Same as input  ParamDataTypeStr=Inherit: Same as input
  IC : Switch  Threshold=Ts  SaturateOnIntegerOverflow=off  InputSameDT=off
  Mux : Mux  Inputs=2
  Prediction : Subsystem
  Sum1 : Sum  Inputs=+-  InputSameDT=on  SaturateOnIntegerOverflow=on  OutDataTypeStr=Inherit: Same as first input
  Sum3 : Sum  InputSameDT=on  SaturateOnIntegerOverflow=on  OutDataTypeStr=Inherit: Same as first input
  Sum9 : Sum  InputSameDT=on  SaturateOnIntegerOverflow=on  OutDataTypeStr=Inherit: Same as first input
  Terminator : Terminator
  sum : Sum  SaturateOnIntegerOverflow=on
  deltat_n : Outport  InitialOutput=0
  "Ts_n " : Outport  Port=2  InitialOutput=0
  dw : Outport  Port=3  InitialOutput=0
  wires:
  Prediction/1(O) -> deltat_n/1
  Demux1/1 -> Terminator/1
  Demux1/2 -> Prediction/1(I)
  Demux/2 -> Sum1/1  "x2(k)"
  Demux/1 -> dw/1  "x1(k)"
  IC/1 -> Demux/1, Delay_x/1
  Sum3/1 -> IC/1  "x(k)"
  Digital Clock/1 -> IC/2
  Delay_x/1 -> Ad*x(k-1)/1, Demux1/1, IC/3  "x(k-1)"
  Ad*x(k-1)/1 -> Sum3/1
  Bd*(u(k)+ u(k-1))/1 -> Sum3/2
  sum/1 -> Bd*(u(k)+ u(k-1))/1  "u(k) + u(k-1)"
  Delay_u/1 -> sum/2
  Tt_n/1 -> Sum9/2
  Ts_n+1/1 -> Sum9/1
  Sum9/1 -> Mux/1  "u1 (k)"
  deltat_n-1/1 -> Sum1/2, Mux/2  "u2(k)"
  Mux/1 -> sum/1, Delay_u/1  "u(k)"
  Sum1/1 -> Gain11/1
  Gain11/1 -> "Ts_n "/1

== system myLibrary/SG_step/Governor-Turbine/Steam Turbine and Governor/Model/4 mass shaft/3 masses/Mass2 ==
  note: implements discretized state-space model of mass dynamic equations using trapezoidal method
      |
      | x(k)= Ad*x(k-1) + Bd*(u(k)+u(k-1))
  note: In order to avoid an algebraic loop
      | the deltat_n(k-1) value is sent to output 1
      | instead of  deltat_n(k).
      | The delay is then compensated by a
      | linear extrapolatiom (Prediction bloc)
  note: Initialization of this delay is not required
      | because x(k) is initialized by IC switch block
  Ts_n+1 : Inport
  Tt_n : Inport  Port=2
  deltat_n-1 : Inport  Port=3
  Ad*x(k-1) : Gain  Gain=Ad  Multiplication=Matrix(K*u)  SaturateOnIntegerOverflow=on  SampleTime=Ts  OutDataTypeStr=Inherit: Same as input  ParamDataTypeStr=Inherit: Same as input
  Bd*(u(k)+ u(k-1)) : Gain  Gain=Bd  Multiplication=Matrix(K*u)  SaturateOnIntegerOverflow=on  SampleTime=Ts  OutDataTypeStr=Inherit: Same as input  ParamDataTypeStr=Inherit: Same as input
  Delay_u : UnitDelay  SampleTime=Ts  HasFrameUpgradeWarning=on
  Delay_x : UnitDelay  InitialCondition=[0 dth0]  SampleTime=Ts  HasFrameUpgradeWarning=on
  Demux : Demux  Outputs=2
  Demux1 : Demux  Outputs=2
  Digital Clock : DigitalClock  SampleTime=Ts
  Gain11 : Gain  Gain=K  SaturateOnIntegerOverflow=on  OutDataTypeStr=Inherit: Same as input  ParamDataTypeStr=Inherit: Same as input
  IC : Switch  Threshold=Ts  SaturateOnIntegerOverflow=off  InputSameDT=off
  Mux : Mux  Inputs=2
  Prediction : Subsystem
  Sum1 : Sum  Inputs=+-  InputSameDT=on  SaturateOnIntegerOverflow=on  OutDataTypeStr=Inherit: Same as first input
  Sum3 : Sum  InputSameDT=on  SaturateOnIntegerOverflow=on  OutDataTypeStr=Inherit: Same as first input
  Sum9 : Sum  InputSameDT=on  SaturateOnIntegerOverflow=on  OutDataTypeStr=Inherit: Same as first input
  Terminator : Terminator
  sum : Sum  SaturateOnIntegerOverflow=on
  deltat_n : Outport  InitialOutput=0
  "Ts_n " : Outport  Port=2  InitialOutput=0
  dw : Outport  Port=3  InitialOutput=0
  wires:
  Prediction/1(O) -> deltat_n/1
  Demux1/1 -> Terminator/1
  Demux1/2 -> Prediction/1(I)
  Demux/2 -> Sum1/1  "x2(k)"
  Demux/1 -> dw/1  "x1(k)"
  IC/1 -> Demux/1, Delay_x/1
  Sum3/1 -> IC/1  "x(k)"
  Digital Clock/1 -> IC/2
  Delay_x/1 -> Ad*x(k-1)/1, Demux1/1, IC/3  "x(k-1)"
  Ad*x(k-1)/1 -> Sum3/1
  Bd*(u(k)+ u(k-1))/1 -> Sum3/2
  sum/1 -> Bd*(u(k)+ u(k-1))/1  "u(k) + u(k-1)"
  Delay_u/1 -> sum/2
  Tt_n/1 -> Sum9/2
  Ts_n+1/1 -> Sum9/1
  Sum9/1 -> Mux/1  "u1 (k)"
  deltat_n-1/1 -> Sum1/2, Mux/2  "u2(k)"
  Mux/1 -> sum/1, Delay_u/1  "u(k)"
  Sum1/1 -> Gain11/1
  Gain11/1 -> "Ts_n "/1
